simulink model "RmtAPP_PlausBrk"  (R2016b)
settings: configuration reference "CodeGenConfigSet" (kept outside this file)
values from neighbouring files (symbols this model uses):
  RmtAPP_drUnFltLim_C = Calibration.Parameter    [init_RmtAPP_PlausBrk.m]    (also in init_RmtAPP_PlausBrk_SIL.m = Simulink.Parameter)
  RmtAPP_nLim_C = Calibration.Parameter    [init_RmtAPP_PlausBrk.m]    (also in init_RmtAPP_PlausBrk_SIL.m = Simulink.Parameter)
  RmtAPP_swtAppGradEna_C = Calibration.Parameter    [init_RmtAPP_PlausBrk.m]    (also in init_RmtAPP_PlausBrk_SIL.m = Simulink.Parameter)
  RmtAPP_swtBrkDet_C = Calibration.Parameter    [init_RmtAPP_PlausBrk.m]    (also in init_RmtAPP_PlausBrk_SIL.m = Simulink.Parameter)
  RmtAPP_swtRstCon_C = Calibration.Parameter    [init_RmtAPP_PlausBrk.m]    (also in init_RmtAPP_PlausBrk_SIL.m = Simulink.Parameter)
  RmtAPP_tiGradCondDebHiLo_C = Calibration.Parameter    [init_RmtAPP_PlausBrk.m]    (also in init_RmtAPP_PlausBrk_SIL.m = Simulink.Parameter)
  RmtAPP_tiGradCondDebLoHi_C = Calibration.Parameter    [init_RmtAPP_PlausBrk.m]    (also in init_RmtAPP_PlausBrk_SIL.m = Simulink.Parameter)
  RmtAPP_tiPlaBrkDetDeb_C = Calibration.Parameter    [init_RmtAPP_PlausBrk.m]    (also in init_RmtAPP_PlausBrk_SIL.m = Simulink.Parameter)
  RmtAPP_tiPlaBrkRstDeb_C = Calibration.Parameter    [init_RmtAPP_PlausBrk.m]    (also in init_RmtAPP_PlausBrk_SIL.m = Simulink.Parameter)
  RmtAPP_vLim_C = Calibration.Parameter    [init_RmtAPP_PlausBrk.m]    (also in init_RmtAPP_PlausBrk_SIL.m = Simulink.Parameter)
undefined symbols (not defined in the file or in its folder): AccPedal_switch_conv, RmtAPP_PlausBrk_DT, Switch_conv
libraries: CXLib x9
settings Model: Creator=bianxuyin  LastModifiedBy=bianxuyin
settings ConfigSetRef: SourceLocation=Base Workspace

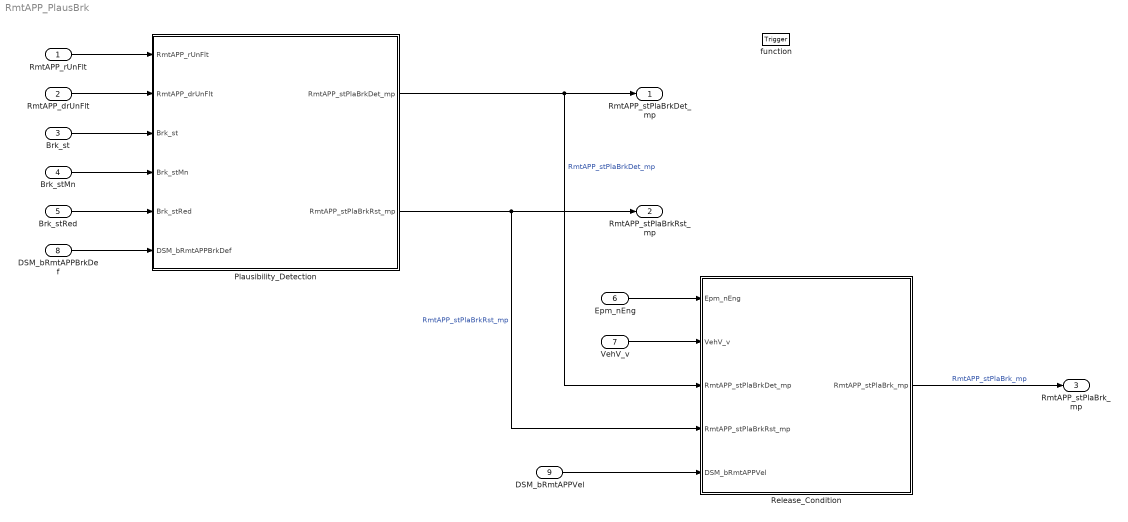
== system RmtAPP_PlausBrk ==
  RmtAPP_rUnFlt : Inport  Tag=%  Description=Unfiltered RmtAPP value  OutMin=0  OutMax=100  OutDataTypeStr=Accpedal_rate
  RmtAPP_drUnFlt : Inport  Tag=%/s  Description=Remote Acceleration pedal position gradient of unfilterd value  Port=2  OutMin=-100000  OutMax=100000  OutDataTypeStr=Accpedal_rate_s
  Brk_st : Inport  Description=Brake switch state  Port=3  OutMin=0  OutMax=255  OutDataTypeStr=State_uint8
  Brk_stMn : Inport  Description=Status of the main brake  Port=4  OutMin=0  OutMax=1  OutDataTypeStr=boolean
  Brk_stRed : Inport  Description=Status of the redundant break  Port=5  OutMin=0  OutMax=1  OutDataTypeStr=boolean
  Epm_nEng : Inport  Tag=rpm  Description=Engine speed  Port=6  OutMin=0  OutMax=6000  OutDataTypeStr=EngSpeed_rpm
  VehV_v : Inport  Tag=km/h  Description=Vehicle speed  Port=7  OutMin=0  OutMax=250  OutDataTypeStr=VehSpeed_km_h
  DSM_bRmtAPPBrkDef : Inport  Description=status of FId_RmtAPPBrkDef  Port=8  OutMin=0  OutMax=1  OutDataTypeStr=boolean
  DSM_bRmtAPPVel : Inport  Description=status of FId_RmtAPPVel  Port=9  OutMin=0  OutMax=1  OutDataTypeStr=boolean
  function : TriggerPort  TriggerType=function-call  VariantControl=Variant
  Plausibility_Detection : Subsystem
  Release_Condition : Subsystem
  RmtAPP_stPlaBrkDet_mp : Outport  Description=State of detection plausibility with brake  OutMin=0  OutMax=1  OutDataTypeStr=boolean
  RmtAPP_stPlaBrkRst_mp : Outport  Description=State of reset plausibility with brake  Port=2  OutMin=0  OutMax=1  OutDataTypeStr=boolean
  RmtAPP_stPlaBrk_mp : Outport  Description=State of plausibility RmtAPP with brake  Port=3  OutMin=0  OutMax=1  OutDataTypeStr=boolean
  wires:
  Plausibility_Detection/1(RmtAPP_stPlaBrkDet_mp) -> RmtAPP_stPlaBrkDet_mp/1, Release_Condition/3(RmtAPP_stPlaBrkDet_mp)  "RmtAPP_stPlaBrkDet_mp"
  Plausibility_Detection/2(RmtAPP_stPlaBrkRst_mp) -> Release_Condition/4(RmtAPP_stPlaBrkRst_mp), RmtAPP_stPlaBrkRst_mp/1  "RmtAPP_stPlaBrkRst_mp"
  Release_Condition/1(RmtAPP_stPlaBrk_mp) -> RmtAPP_stPlaBrk_mp/1  "RmtAPP_stPlaBrk_mp"
  RmtAPP_rUnFlt/1 -> Plausibility_Detection/1(RmtAPP_rUnFlt)
  RmtAPP_drUnFlt/1 -> Plausibility_Detection/2(RmtAPP_drUnFlt)
  Brk_st/1 -> Plausibility_Detection/3(Brk_st)
  Brk_stMn/1 -> Plausibility_Detection/4(Brk_stMn)
  Brk_stRed/1 -> Plausibility_Detection/5(Brk_stRed)
  DSM_bRmtAPPBrkDef/1 -> Plausibility_Detection/6(DSM_bRmtAPPBrkDef)
  Epm_nEng/1 -> Release_Condition/1(Epm_nEng)
  VehV_v/1 -> Release_Condition/2(VehV_v)
  DSM_bRmtAPPVel/1 -> Release_Condition/5(DSM_bRmtAPPVel)

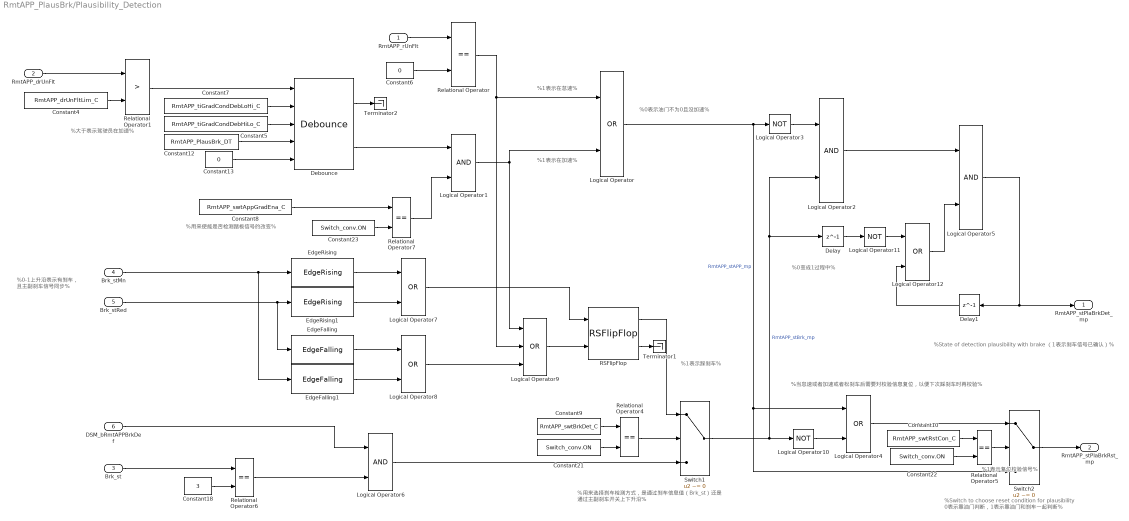
== system RmtAPP_PlausBrk/Plausibility_Detection ==
  note: %用来选择刹车检测方式，是通过刹车信息值（Brk_st）还是
      | 通过主副刹车开关上下升沿%
  note: %用来使能是否检测踏板信号的改变%
  note: %大于表示驾驶员在加速%
  note: %State of detection plausibility with brake（1表示刹车信号已确认）%
  note: %1表示复位校验信号%
  note: %Switch to choose reset condition for plausibility
      | 0表示靠油门判断，1表示靠油门和刹车一起判断%
  note: %0-1上升沿表示有刹车，
      | 且主副刹车信号同步%
  note: %1表示在加速%
  note: %1表示踩刹车%
  note: %当怠速或者加速或者松刹车后需要对校验信息复位，以便下次踩刹车时再校验%
  note: %0变成1过程中%
  note: %0表示油门不为0且没加速%
  note: %1表示在怠速%
  RmtAPP_rUnFlt : Inport  Tag=%  Description=Unfiltered APP value  OutMin=0  OutMax=100  OutDataTypeStr=Accpedal_rate
  RmtAPP_drUnFlt : Inport  Tag=%  Description=Acceleration pedal position gradient of unfilterd value  Port=2  OutMin=-200  OutMax=200  OutDataTypeStr=Accpedal_rate_s
  Brk_st : Inport  Tag=-  Description=Brake switch state  Port=3  OutMin=0  OutMax=255  OutDataTypeStr=State_uint8
  Brk_stMn : Inport  Tag=-  Description=Status of the main brake  Port=4  OutMin=0  OutMax=1  OutDataTypeStr=boolean
  Brk_stRed : Inport  Tag=-  Description=Status of the redundant break  Port=5  OutMin=0  OutMax=1  OutDataTypeStr=boolean
  DSM_bRmtAPPBrkDef : Inport  Tag=-  Description=status of FId_APPBrkDef  Port=6  OutMin=0  OutMax=1  OutDataTypeStr=boolean
  Constant10 : Constant  Value=RmtAPP_swtRstCon_C
  Constant12 : Constant  Value=RmtAPP_PlausBrk_DT  OutDataTypeStr=Inherit: Inherit via back propagation
  Constant13 : Constant  Value=0  OutDataTypeStr=boolean
  Constant18 : Constant  Value=3  OutDataTypeStr=Inherit: Inherit via back propagation
  Constant21 : Constant  Value=Switch_conv.ON  OutDataTypeStr=Inherit: Inherit via back propagation
  Constant22 : Constant  Value=Switch_conv.ON  OutDataTypeStr=Inherit: Inherit via back propagation
  Constant23 : Constant  Value=Switch_conv.ON  OutDataTypeStr=Inherit: Inherit via back propagation
  Constant4 : Constant  Value=RmtAPP_drUnFltLim_C
  Constant5 : Constant  Value=RmtAPP_tiGradCondDebHiLo_C
  Constant6 : Constant  Value=0  OutDataTypeStr=Inherit: Inherit via back propagation
  Constant7 : Constant  Value=RmtAPP_tiGradCondDebLoHi_C
  Constant8 : Constant  Value=RmtAPP_swtAppGradEna_C
  Constant9 : Constant  Value=RmtAPP_swtBrkDet_C
  Debounce : CXLib/Debounce
  Delay : Delay  DelayLength=1  InitialCondition=0
  Delay1 : Delay  DelayLength=1  InitialCondition=0
  EdgeFalling : CXLib/EdgeFalling
  EdgeFalling1 : CXLib/EdgeFalling
  EdgeRising : CXLib/EdgeRising
  EdgeRising1 : CXLib/EdgeRising
  Logical Operator{,4,7..8,12} (5 alike) : Logic  Operator=OR  OutDataTypeStr=boolean
  Logical Operator{1..2,5..6} (4 alike) : Logic  OutDataTypeStr=boolean
  Logical Operator10 : Logic  Operator=NOT  AllPortsSameDT=off  OutDataTypeStr=boolean
  Logical Operator11 : Logic  Operator=NOT  AllPortsSameDT=off  OutDataTypeStr=boolean
  Logical Operator3 : Logic  Operator=NOT  AllPortsSameDT=off  OutDataTypeStr=boolean
  Logical Operator9 : Logic  Operator=OR  Inputs=3  OutDataTypeStr=boolean
  RSFlipFlop : CXLib/RSFlipFlop
  Relational Operator{,4..7} (5 alike) : RelationalOperator  Operator===  OutDataTypeStr=boolean  RndMeth=Nearest  InputSameDT=on
  Relational Operator1 : RelationalOperator  Operator=>  OutDataTypeStr=boolean  RndMeth=Nearest  InputSameDT=on
  Switch1 : Switch  Criteria=u2 ~= 0  Threshold=AccPedal_switch_conv.OFF  InputSameDT=on
  Switch2 : Switch  Criteria=u2 ~= 0  InputSameDT=on
  Terminator1 : Terminator
  Terminator2 : Terminator
  RmtAPP_stPlaBrkDet_mp : Outport  Tag=-  Description=State of detection plausibility with brake  OutMin=0  OutMax=1  OutDataTypeStr=boolean
  RmtAPP_stPlaBrkRst_mp : Outport  Tag=-  Description=State of reset plausibility with brake  Port=2  OutMin=0  OutMax=1  OutDataTypeStr=boolean
  wires:
  Constant23/1 -> Relational Operator7/2
  Constant22/1 -> Relational Operator5/2
  Constant21/1 -> Relational Operator4/2
  Relational Operator4/1 -> Switch1/2
  DSM_bRmtAPPBrkDef/1 -> Logical Operator6/1
  Brk_st/1 -> Relational Operator6/1
  Constant18/1 -> Relational Operator6/2
  Debounce/2 -> Logical Operator1/1
  Constant13/1 -> Debounce/5
  Constant12/1 -> Debounce/4
  Debounce/1 -> Terminator2/1
  Switch2/1 -> RmtAPP_stPlaBrkRst_mp/1
  Logical Operator5/1 -> RmtAPP_stPlaBrkDet_mp/1, Delay1/1
  Relational Operator6/1 -> Logical Operator6/2
  Relational Operator5/1 -> Switch2/2
  Relational Operator7/1 -> Logical Operator1/2
  RSFlipFlop/2 -> Terminator1/1
  Constant10/1 -> Relational Operator5/1
  Logical Operator4/1 -> Switch2/1
  Logical Operator10/1 -> Logical Operator4/2
  Logical Operator12/1 -> Logical Operator5/2
  Delay1/1 -> Logical Operator12/2
  Logical Operator11/1 -> Logical Operator12/1
  Delay/1 -> Logical Operator11/1
  Logical Operator2/1 -> Logical Operator5/1
  Switch1/1 -> Logical Operator10/1, Logical Operator2/2, Delay/1  "RmtAPP_stBrk_mp"
  Logical Operator6/1 -> Switch1/3
  RSFlipFlop/1 -> Switch1/1
  Logical Operator9/1 -> RSFlipFlop/2
  Logical Operator7/1 -> RSFlipFlop/1
  Logical Operator8/1 -> Logical Operator9/3
  EdgeFalling1/1 -> Logical Operator8/2
  EdgeFalling/1 -> Logical Operator8/1
  EdgeRising1/1 -> Logical Operator7/2
  EdgeRising/1 -> Logical Operator7/1
  Brk_stRed/1 -> EdgeRising1/1, EdgeFalling/1
  Brk_stMn/1 -> EdgeRising/1, EdgeFalling1/1
  Constant9/1 -> Relational Operator4/1
  Logical Operator3/1 -> Logical Operator2/1
  Logical Operator/1 -> Logical Operator3/1, Switch2/3, Logical Operator4/1  "RmtAPP_stAPP_mp"
  Logical Operator1/1 -> Logical Operator/2, Logical Operator9/1
  Constant8/1 -> Relational Operator7/1
  Constant5/1 -> Debounce/3
  Constant7/1 -> Debounce/2
  Relational Operator1/1 -> Debounce/1
  Constant6/1 -> Relational Operator/2
  Relational Operator/1 -> Logical Operator9/2, Logical Operator/1
  Constant4/1 -> Relational Operator1/2
  RmtAPP_drUnFlt/1 -> Relational Operator1/1
  RmtAPP_rUnFlt/1 -> Relational Operator/1

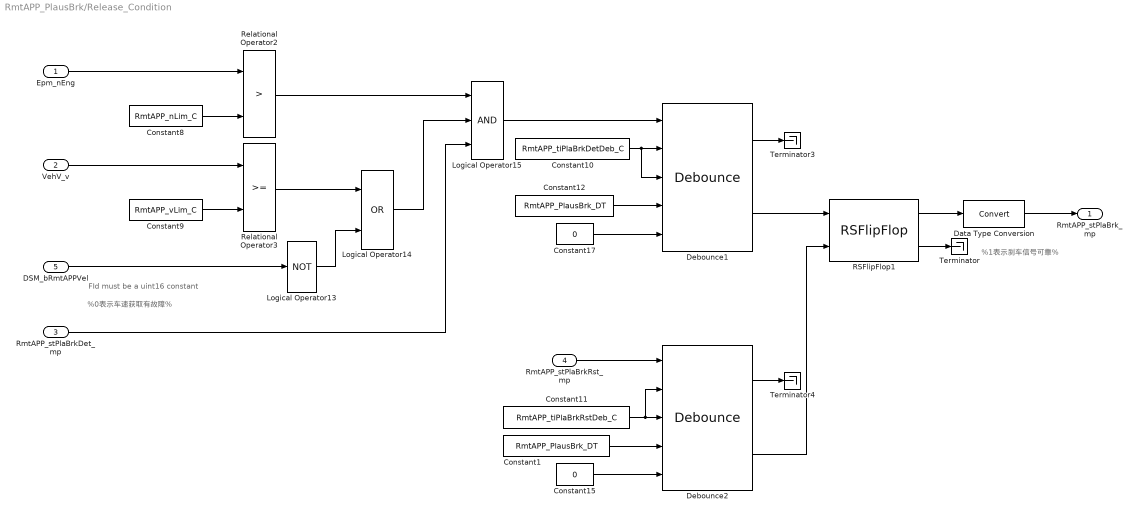
== system RmtAPP_PlausBrk/Release_Condition ==
  note: FId must be a uint16 constant
  note: %1表示刹车信号可靠%
  note: %0表示车速获取有故障%
  Epm_nEng : Inport
  VehV_v : Inport  Port=2
  RmtAPP_stPlaBrkDet_mp : Inport  Port=3
  RmtAPP_stPlaBrkRst_mp : Inport  Port=4
  DSM_bRmtAPPVel : Inport  Tag=-  Description=status of FId_APPVel  Port=5  OutMin=0  OutMax=1
  Constant1 : Constant  Value=RmtAPP_PlausBrk_DT  OutDataTypeStr=Inherit: Inherit via back propagation
  Constant10 : Constant  Value=RmtAPP_tiPlaBrkDetDeb_C
  Constant11 : Constant  Value=RmtAPP_tiPlaBrkRstDeb_C
  Constant12 : Constant  Value=RmtAPP_PlausBrk_DT  OutDataTypeStr=Inherit: Inherit via back propagation
  Constant15 : Constant  Value=0  OutDataTypeStr=boolean
  Constant17 : Constant  Value=0  OutDataTypeStr=boolean
  Constant8 : Constant  Value=RmtAPP_nLim_C
  Constant9 : Constant  Value=RmtAPP_vLim_C
  Data Type Conversion : DataTypeConversion
  Debounce1 : CXLib/Debounce  RequirementInfo={'other' 'APP_requirements.doc' '@Simulink_requirement_item_18' 'true' '刹车校验使能条件。' '' } %GIDa_b2158508_3669_4b5a_a44f_72e92b93bfae
  Debounce2 : CXLib/Debounce  RequirementInfo={'other' 'APP_requirements.doc' '@Simulink_requirement_item_17' 'true' '刹车校验结果复位。' '' ; 'other' 'APP_requirements.doc' '@Simulink_requirement_item_18' 'true' '刹车校验使能条件。' '' } %GIDa_b68598b8_2e9a_4630_8ab0_46ad845c33bd
  Logical Operator13 : Logic  Operator=NOT  AllPortsSameDT=off  OutDataTypeStr=boolean
  Logical Operator14 : Logic  Operator=OR  OutDataTypeStr=boolean
  Logical Operator15 : Logic  Inputs=3  OutDataTypeStr=boolean
  RSFlipFlop1 : CXLib/RSFlipFlop
  Relational Operator2 : RelationalOperator  Operator=>  OutDataTypeStr=boolean  RndMeth=Nearest  InputSameDT=on
  Relational Operator3 : RelationalOperator  OutDataTypeStr=boolean  RndMeth=Nearest  InputSameDT=on
  Terminator : Terminator
  Terminator3 : Terminator
  Terminator4 : Terminator
  RmtAPP_stPlaBrk_mp : Outport
  wires:
  RmtAPP_stPlaBrkRst_mp/1 -> Debounce2/1
  RmtAPP_stPlaBrkDet_mp/1 -> Logical Operator15/3
  Logical Operator13/1 -> Logical Operator14/2
  Data Type Conversion/1 -> RmtAPP_stPlaBrk_mp/1
  RSFlipFlop1/1 -> Data Type Conversion/1
  DSM_bRmtAPPVel/1 -> Logical Operator13/1
  Debounce2/1 -> Terminator4/1
  Constant17/1 -> Debounce1/5
  Constant12/1 -> Debounce1/4
  Debounce1/1 -> Terminator3/1
  Constant15/1 -> Debounce2/5
  Constant1/1 -> Debounce2/4
  Constant8/1 -> Relational Operator2/2
  Constant9/1 -> Relational Operator3/2
  RSFlipFlop1/2 -> Terminator/1
  Debounce2/2 -> RSFlipFlop1/2
  Constant11/1 -> Debounce2/2, Debounce2/3
  Debounce1/2 -> RSFlipFlop1/1
  Constant10/1 -> Debounce1/3, Debounce1/2
  Logical Operator15/1 -> Debounce1/1
  Logical Operator14/1 -> Logical Operator15/2
  Relational Operator2/1 -> Logical Operator15/1
  Relational Operator3/1 -> Logical Operator14/1
  VehV_v/1 -> Relational Operator3/1
  Epm_nEng/1 -> Relational Operator2/1
